simulink library "EmE_MBD_Blockset"  (R2018a)
settings: Solver=ode1  StartTime=0.0  StopTime=Inf  FixedStep=0.001  RelTol=1e-3  EnableMultiTasking=on
PostLoadFcn:
  | , if any(exist('dsrtsu_mdlpostloadfcn', 'file') == [2, 3, 6]), try dsrtsu_mdlpostloadfcn('Execute', bdroot); catch fprintf('Error in PostLoadFcn (dsrtsu_mdlpostloadfcn) for model "%s":\n %s\n', bdroot, lasterr); end, end,
undefined symbols (not defined in the file or in its folder): ENUM_TSC1_CONTROL_PURPOSE_T, gcbh, GLB_SWITCH_T
libraries: simulink x237, $bdroot x115, simulink_need_slupdate x26, MotoHawk_lib x13, simulink_extras x3
(part 4 of 11)

== system EmE_MBD_Blockset/Math Operators/Normalize_on_min_max ==
  Max : Inport
  In : Inport  Port=2
  Min : Inport  Port=3
  Constant : Constant  Value=true
  Divide1 : Product  Inputs=*/  InputSameDT=on
  Divide2 : Product  Inputs=*/  InputSameDT=on
  Dynamic_saturation : $bdroot/Discontinuities/Dynamic_saturation
  If_Then_Else : $bdroot/Signal Routing/If_Then_Else
  Subtract1 : Sum  Inputs=+-  InputSameDT=on
  Subtract3 : Sum  Inputs=+-  InputSameDT=on
  Subtract4 : Sum  Inputs=-+  InputSameDT=on
  Norm : Outport  LibraryBlock=$bdroot/Sinks/Out  OutputWhenDisabled=reset
  wires:
  Dynamic_saturation/1 -> Subtract1/2, Subtract3/1
  Max/1 -> Dynamic_saturation/1, Subtract4/2, Subtract1/1
  Min/1 -> Dynamic_saturation/3, Subtract4/1, Subtract3/2
  Subtract1/1 -> Divide1/1
  Subtract4/1 -> Divide1/2, Divide2/2
  In/1 -> Dynamic_saturation/2
  Subtract3/1 -> Divide2/1
  Constant/1 -> If_Then_Else/1
  Divide2/1 -> If_Then_Else/2  "norm_on_min"
  Divide1/1 -> If_Then_Else/3  "norm_on_max"
  If_Then_Else/1 -> Norm/1

== system EmE_MBD_Blockset/Math Operators/Slew ==
  In : Inport
  Inc : Inport  Port=2
  Dec : Inport  Port=3
  dT : Inport  Port=4
  Abs : $bdroot/Math Operators/Abs
  Abs1 : $bdroot/Math Operators/Abs
  Add1 : Sum  InputSameDT=on
  Check Static Lower Bound : simulink/Model Verification/Check Static  Lower Bound  Description=0 <= u  min=0  min_included=on  enabled=on  stopWhenAssertionFail=on  export=off  icon=graphic
      settings: SourceProductName=Simulink
  MinMax1 : MinMax  Function=max  Inputs=2  InputSameDT=on
  MinMax2 : MinMax  Inputs=2  InputSameDT=on
  Product1 : Product  InputSameDT=on
  Product2 : Product  InputSameDT=on
  Subtract1 : Sum  Inputs=+-  InputSameDT=on
  Unit Delay External IC : simulink_need_slupdate/Unit Delay External IC  tsamp=-1
      settings: SourceProductName=Simulink  SourceProductBaseCode=SL
  Out : Outport
  wires:
  Add1/1 -> MinMax2/2
  Subtract1/1 -> MinMax1/2
  MinMax1/1 -> Out/1, Unit Delay External IC/1
  Product1/1 -> Add1/2
  Unit Delay External IC/1 -> Subtract1/1, Add1/1
  Dec/1 -> Abs1/1
  MinMax2/1 -> MinMax1/1
  Inc/1 -> Check Static Lower Bound/1, Abs/1
  In/1 -> MinMax2/1, Unit Delay External IC/2
  Product2/1 -> Subtract1/2
  Abs/1 -> Product1/1
  Abs1/1 -> Product2/2
  dT/1 -> Product2/1, Product1/2

== system EmE_MBD_Blockset/Math Operators/Slew_at_event ==
  F_Event_trigger : Inport
  Init : Inport  Port=2
  In : Inport  Port=3
  Inc : Inport  Port=4
  Dec : Inport  Port=5
  dT : Inport  Port=6
  Enable : EnablePort  StatesWhenEnabling=reset
  Abs : Abs
  Constant1 : Constant
  RS flip-flop : $bdroot/Logic and Bit Operations/RS flip-flop
  Relational Operator1 : $bdroot/Logic and Bit Operations/Relational Operator  func=<=
  Rising_edge : $bdroot/Discontinuities/Rising_edge  initact=off
      settings: AttributesFormatString=Action on IC: %<initact>
  Slew_init_reset : $bdroot/Math Operators/Slew_init_reset
  Subtract : Sum  Inputs=-+  InputSameDT=on
  Terminator : Terminator
  F_Out_slewing : Outport  OutputWhenDisabled=reset  InitialOutput=false
      settings: AttributesFormatString=IC: %<InitialOutput>\nDisabled value: %<OutputWhenDisabled>
  Out : Outport  Port=2  OutputWhenDisabled=reset  InitialOutput=single(0)
      settings: AttributesFormatString=IC: %<InitialOutput>\nDisabled value: %<OutputWhenDisabled>
  wires:
  RS flip-flop/2 -> Terminator/1
  RS flip-flop/1 -> F_Out_slewing/1  "F_Value_slew_enabled"
  Relational Operator1/1 -> RS flip-flop/1
  Constant1/1 -> Relational Operator1/2
  Subtract/1 -> Abs/1
  Abs/1 -> Relational Operator1/1
  In/1 -> Slew_init_reset/3, Subtract/2
  Init/1 -> Slew_init_reset/2
  Rising_edge/1 -> Slew_init_reset/1
  F_Event_trigger/1 -> Rising_edge/1, RS flip-flop/2
  dT/1 -> Slew_init_reset/6
  Dec/1 -> Slew_init_reset/5
  Inc/1 -> Slew_init_reset/4
  Slew_init_reset/1 -> Subtract/1, Out/1  "Value_slewed"

== system EmE_MBD_Blockset/Math Operators/Slew_init_reset ==
  F_Reset : Inport
  Init : Inport  Port=2
  In : Inport  Port=3
  Inc : Inport  Port=4
  Dec : Inport  Port=5
  dT : Inport  Port=6
  Abs : $bdroot/Math Operators/Abs
  Abs1 : $bdroot/Math Operators/Abs
  Add1 : Sum  InputSameDT=on
  Check Static Lower Bound : simulink/Model Verification/Check Static  Lower Bound  Description=0 <= u  min=0  min_included=on  enabled=on  stopWhenAssertionFail=on  export=off  icon=graphic
      settings: SourceProductName=Simulink
  Constant : Constant  Value=false
  If_Then_Else : $bdroot/Signal Routing/If_Then_Else
  Logical Operator1 : $bdroot/Logic and Bit Operations/Logical Operator  Operator=OR  Inputs=2
  MinMax1 : MinMax  Function=max  Inputs=2  InputSameDT=on
  MinMax2 : MinMax  Inputs=2  InputSameDT=on
  Product1 : Product  InputSameDT=on
  Product2 : Product  InputSameDT=on
  Subtract1 : Sum  Inputs=+-  InputSameDT=on
  Unit Delay External IC : simulink_need_slupdate/Unit Delay External IC  tsamp=-1
      settings: SourceProductName=Simulink  SourceProductBaseCode=SL
  Unit_Delay : UnitDelay  InitialCondition=true  SampleTime=-1
      settings: AttributesFormatString=IC: %<vinit>
  Out : Outport
  wires:
  MinMax2/1 -> MinMax1/1
  Product1/1 -> Add1/2
  MinMax1/1 -> If_Then_Else/3
  In/1 -> MinMax2/1, Unit Delay External IC/2
  Product2/1 -> Subtract1/2
  Add1/1 -> MinMax2/2
  Subtract1/1 -> MinMax1/2
  Unit Delay External IC/1 -> Subtract1/1, Add1/1
  Inc/1 -> Check Static Lower Bound/1, Abs/1
  Dec/1 -> Abs1/1
  dT/1 -> Product2/1, Product1/2
  Unit_Delay/1 -> Logical Operator1/2
  Init/1 -> If_Then_Else/2
  F_Reset/1 -> Logical Operator1/1
  Logical Operator1/1 -> If_Then_Else/1
  If_Then_Else/1 -> Unit Delay External IC/1, Out/1
  Constant/1 -> Unit_Delay/1
  Abs1/1 -> Product2/2
  Abs/1 -> Product1/1

== system EmE_MBD_Blockset/Math Operators/Slope_intercept ==
  X1 : Inport
  X2 : Inport  Port=2
  Y1 : Inport  Port=3
  Y2 : Inport  Port=4
  Compare To Zero : simulink/Logic and Bit Operations/Compare To Zero  relop===  OutDataTypeStr=boolean
  Constant10 : Constant  Value=0.0001
  Divide : Product  Inputs=*/  InputSameDT=on
  If_Then_Else : $bdroot/Signal Routing/If_Then_Else
  Product : Product  InputSameDT=on
  Subtract : Sum  Inputs=+-  InputSameDT=on
  Subtract1 : Sum  Inputs=+-  InputSameDT=on
  Subtract2 : Sum  Inputs=+-  InputSameDT=on
  m : Outport  OutputWhenDisabled=reset  InitialOutput=0
  b : Outport  Port=2  OutputWhenDisabled=reset  InitialOutput=0
  wires:
  Subtract2/1 -> b/1
  Divide/1 -> Product/1, m/1
  Subtract/1 -> Divide/1
  Subtract1/1 -> If_Then_Else/3, Compare To Zero/1
  Product/1 -> Subtract2/2
  Y2/1 -> Subtract/1
  X1/1 -> Subtract1/2, Product/2
  Y1/1 -> Subtract/2, Subtract2/1
  X2/1 -> Subtract1/1
  Compare To Zero/1 -> If_Then_Else/1
  Constant10/1 -> If_Then_Else/2
  If_Then_Else/1 -> Divide/2

== system EmE_MBD_Blockset/Math Operators/Soft_transition ==
  In : Inport
  T_Inc : Inport  Port=2
  T_Dec : Inport  Port=3
  Abs2 : $bdroot/Math Operators/Abs
  CPV : $bdroot/Sources/CPV  conval=false
  Detect Change : simulink/Logic and Bit Operations/Detect Change  vinit=0  InputProcessing=Inherited  OutDataTypeStr=boolean
      settings: AttributesFormatString=IC: %<vinit>
  Divide1 : Product  Inputs=*/  InputSameDT=on
  Divide2 : Product  Inputs=*/  InputSameDT=on
  If_Then_Else2 : $bdroot/Signal Routing/If_Then_Else
  If_Then_Else3 : $bdroot/Signal Routing/If_Then_Else
  MinMax : MinMax  Function=max  Inputs=2  InputSameDT=on
  MinMax1 : MinMax  Function=max  Inputs=2  InputSameDT=on
  Saturation : Saturate  UpperLimit=Inf  LowerLimit=0.0001
      settings: AttributesFormatString=%<LowerLimit>-%<UpperLimit>
  Saturation1 : Saturate  UpperLimit=Inf  LowerLimit=0.0001
      settings: AttributesFormatString=%<LowerLimit>-%<UpperLimit>
  Slew_init_reset : $bdroot/Math Operators/Slew_init_reset
  Subtract : Sum  Inputs=+-  InputSameDT=on
  Unit Delay External IC2 : simulink_need_slupdate/Unit Delay External IC  tsamp=-1
      settings: SourceProductName=Simulink  SourceProductBaseCode=SL
  Unit Delay External IC3 : simulink_need_slupdate/Unit Delay External IC  tsamp=-1
      settings: SourceProductName=Simulink  SourceProductBaseCode=SL
  Unit_Delay : UnitDelay  SampleTime=-1
      settings: AttributesFormatString=IC: %<vinit>
  dT : $bdroot/Sources/dT
  Out : Outport  OutputWhenDisabled=reset
  wires:
  Slew_init_reset/1 -> Unit_Delay/1, Out/1
  CPV/1 -> Slew_init_reset/1
  dT/1 -> MinMax1/2, MinMax/2, Slew_init_reset/6
  Unit_Delay/1 -> [Out_prev]
  In/1 -> Slew_init_reset/3, Slew_init_reset/2, Detect Change/1, Subtract/2
  [Out_prev] -> Subtract/1
  Subtract/1 -> Abs2/1  "err"
  Detect Change/1 -> If_Then_Else3/1, If_Then_Else2/1
  Unit Delay External IC3/1 -> If_Then_Else3/3
  Divide1/1 -> Unit Delay External IC3/2, If_Then_Else3/2
  If_Then_Else3/1 -> Slew_init_reset/5, Unit Delay External IC3/1
  T_Inc/1 -> MinMax/1
  Unit Delay External IC2/1 -> If_Then_Else2/3
  Divide2/1 -> Unit Delay External IC2/2, If_Then_Else2/2
  If_Then_Else2/1 -> Unit Delay External IC2/1, Slew_init_reset/4
  Saturation/1 -> Divide2/2
  Saturation1/1 -> Divide1/2
  Abs2/1 -> Divide1/1, Divide2/1  "err_abs"
  MinMax/1 -> Saturation/1
  MinMax1/1 -> Saturation1/1
  T_Dec/1 -> MinMax1/1

== system EmE_MBD_Blockset/Obsolete/Normalize_on_max ==
  Max : Inport
  In : Inport  Port=2
  Min : Inport  Port=3
  Divide1 : Product  Inputs=*/  InputSameDT=on
  Dynamic_saturation : $bdroot/Discontinuities/Dynamic_saturation
  Subtract1 : Sum  Inputs=+-  InputSameDT=on
  Subtract2 : Sum  Inputs=-+  InputSameDT=on
  Norm : Outport  LibraryBlock=$bdroot/Sinks/Out  OutputWhenDisabled=reset
  wires:
  Max/1 -> Subtract1/1, Dynamic_saturation/1, Subtract2/2
  Min/1 -> Subtract2/1, Dynamic_saturation/3
  Divide1/1 -> Norm/1
  Dynamic_saturation/1 -> Subtract1/2
  In/1 -> Dynamic_saturation/2
  Subtract1/1 -> Divide1/1
  Subtract2/1 -> Divide1/2

== system EmE_MBD_Blockset/Obsolete/Normalize_on_min ==
  Max : Inport
  In : Inport  Port=2
  Min : Inport  Port=3
  Divide2 : Product  Inputs=*/  InputSameDT=on
  Dynamic_saturation : $bdroot/Discontinuities/Dynamic_saturation
  Subtract3 : Sum  Inputs=+-  InputSameDT=on
  Subtract4 : Sum  Inputs=-+  InputSameDT=on
  Norm : Outport  LibraryBlock=$bdroot/Sinks/Out  OutputWhenDisabled=reset
  wires:
  In/1 -> Dynamic_saturation/2
  Min/1 -> Dynamic_saturation/3, Subtract4/1, Subtract3/2
  Subtract4/1 -> Divide2/2
  Dynamic_saturation/1 -> Subtract3/1
  Max/1 -> Subtract4/2, Dynamic_saturation/1
  Divide2/1 -> Norm/1
  Subtract3/1 -> Divide2/1

== system EmE_MBD_Blockset/Ports and Subsystems/Enabled Subsystem ==
  In : Inport
  Enable : EnablePort  StatesWhenEnabling=reset
      settings: AttributesFormatString=States when enabling: %<StatesWhenEnabling>
      settings: CopyFcn=|
      | try
      | L = find_system(get(gcbh,'Parent'),'BlockType','Outport');
      | M = find_system(get(gcbh,'Parent'),'BlockType','EnablePort');
      | N = find_system(get(gcbh,'Parent'),'BlockType','TriggerPort');
      | anyoutports = ~isempty(L);
      | anyenableports = ~isempty(M);
      | anytriggerports = ~isempty(N);
      | sys = get_param(L,'Handle');
      | noutports = length(sys);
      | if (anyoutports),
      | for i = 1:noutports,
      | set(sys{i},'AttributesFormatString','IC: %<InitialOutput>\nDisabled value: %<OutputWhenDisabled>')
      | end;
      | end;
      | catch
      | end;
      settings: DeleteFcn=|
      | try
      | L = find_system(get(gcbh,'Parent'),'BlockType','Outport');
      | M = find_system(get(gcbh,'Parent'),'BlockType','EnablePort');
      | N = find_system(get(gcbh,'Parent'),'BlockType','TriggerPort');
      | anyoutports = ~isempty(L);
      | anyenableports = ~isempty(M);
      | anytriggerports = ~isempty(N);
      | sys = get_param(L,'Handle');
      | noutports = length(sys);
      | if ((anyoutports) && (~anytriggerports)),
      | for i = 1:noutports,
      | set(sys{i},'AttributesFormatString','')
      | end;
      | end;
      | catch
      | end;
      settings: NameChangeFcn=|
      | try
      | L = find_system(get(gcbh,'Parent'),'BlockType','Outport');
      | M = find_system(get(gcbh,'Parent'),'BlockType','EnablePort');
      | N = find_system(get(gcbh,'Parent'),'BlockType','TriggerPort');
      | anyoutports = ~isempty(L);
      | anyenableports = ~isempty(M);
      | anytriggerports = ~isempty(N);
      | sys = get_param(L,'Handle');
      | noutports = length(sys);
      | if (anyoutports),
      | for i = 1:noutports,
      | set(sys{i},'AttributesFormatString','IC: %<InitialOutput>\nDisabled value: %<OutputWhenDisabled>')
      | end;
      | end;
      | catch
      | end
      settings: MoveFcn=|
      | try
      | L = find_system(get(gcbh,'Parent'),'BlockType','Outport');
      | M = find_system(get(gcbh,'Parent'),'BlockType','EnablePort');
      | N = find_system(get(gcbh,'Parent'),'BlockType','TriggerPort');
      | anyoutports = ~isempty(L);
      | anyenableports = ~isempty(M);
      | anytriggerports = ~isempty(N);
      | sys = get_param(L,'Handle');
      | noutports = length(sys);
      | if (anyoutports),
      | for i = 1:noutports,
      | set(sys{i},'AttributesFormatString','IC: %<InitialOutput>\nDisabled value: %<OutputWhenDisabled>')
      | end;
      | end;
      | catch
      | end;
  Out : Outport  LibraryBlock=$bdroot/Sinks/Out  OutputWhenDisabled=reset
      settings: AttributesFormatString=IC: %<InitialOutput>\nDisabled value: %<OutputWhenDisabled>
  wires:
  In/1 -> Out/1

== system EmE_MBD_Blockset/Ports and Subsystems/Enabled and Triggered Subsystem ==
  In : Inport
  Enable : EnablePort  StatesWhenEnabling=reset
      settings: AttributesFormatString=States when enabling: %<StatesWhenEnabling>
      settings: CopyFcn=|
      | try
      | L = find_system(get(gcbh,'Parent'),'BlockType','Outport');
      | M = find_system(get(gcbh,'Parent'),'BlockType','EnablePort');
      | N = find_system(get(gcbh,'Parent'),'BlockType','TriggerPort');
      | anyoutports = ~isempty(L);
      | anyenableports = ~isempty(M);
      | anytriggerports = ~isempty(N);
      | sys = get_param(L,'Handle');
      | noutports = length(sys);
      | if (anyoutports),
      | for i = 1:noutports,
      | set(sys{i},'AttributesFormatString','IC: %<InitialOutput>\nDisabled value: %<OutputWhenDisabled>')
      | end;
      | end;
      | catch
      | end;
      settings: DeleteFcn=|
      | try
      | L = find_system(get(gcbh,'Parent'),'BlockType','Outport');
      | M = find_system(get(gcbh,'Parent'),'BlockType','EnablePort');
      | N = find_system(get(gcbh,'Parent'),'BlockType','TriggerPort');
      | anyoutports = ~isempty(L);
      | anyenableports = ~isempty(M);
      | anytriggerports = ~isempty(N);
      | sys = get_param(L,'Handle');
      | noutports = length(sys);
      | if ((anyoutports) && (~anytriggerports)),
      | for i = 1:noutports,
      | set(sys{i},'AttributesFormatString','')
      | end;
      | end;
      | catch
      | end;
      settings: NameChangeFcn=|
      | try
      | L = find_system(get(gcbh,'Parent'),'BlockType','Outport');
      | M = find_system(get(gcbh,'Parent'),'BlockType','EnablePort');
      | N = find_system(get(gcbh,'Parent'),'BlockType','TriggerPort');
      | anyoutports = ~isempty(L);
      | anyenableports = ~isempty(M);
      | anytriggerports = ~isempty(N);
      | sys = get_param(L,'Handle');
      | noutports = length(sys);
      | if (anyoutports),
      | for i = 1:noutports,
      | set(sys{i},'AttributesFormatString','IC: %<InitialOutput>\nDisabled value: %<OutputWhenDisabled>')
      | end;
      | end;
      | catch
      | end
      settings: MoveFcn=|
      | try
      | L = find_system(get(gcbh,'Parent'),'BlockType','Outport');
      | M = find_system(get(gcbh,'Parent'),'BlockType','EnablePort');
      | N = find_system(get(gcbh,'Parent'),'BlockType','TriggerPort');
      | anyoutports = ~isempty(L);
      | anyenableports = ~isempty(M);
      | anytriggerports = ~isempty(N);
      | sys = get_param(L,'Handle');
      | noutports = length(sys);
      | if (anyoutports),
      | for i = 1:noutports,
      | set(sys{i},'AttributesFormatString','IC: %<InitialOutput>\nDisabled value: %<OutputWhenDisabled>')
      | end;
      | end;
      | catch
      | end;
  Trigger : TriggerPort  VariantControl=(inherit)
      settings: AttributesFormatString=States when enabling: %<StatesWhenEnabling>
      settings: CopyFcn=|
      | try
      | L = find_system(get(gcbh,'Parent'),'BlockType','Outport');
      | M = find_system(get(gcbh,'Parent'),'BlockType','EnablePort');
      | N = find_system(get(gcbh,'Parent'),'BlockType','TriggerPort');
      | anyoutports = ~isempty(L);
      | anyenableports = ~isempty(M);
      | anytriggerports = ~isempty(N);
      | sys = get_param(L,'Handle');
      | noutports = length(sys);
      | if (anyoutports),
      | for i = 1:noutports,
      | set(sys{i},'AttributesFormatString','IC: %<InitialOutput>\nDisabled value: %<OutputWhenDisabled>')
      | end;
      | end;
      | catch
      | end;
      settings: DeleteFcn=|
      | try
      | L = find_system(get(gcbh,'Parent'),'BlockType','Outport');
      | M = find_system(get(gcbh,'Parent'),'BlockType','EnablePort');
      | N = find_system(get(gcbh,'Parent'),'BlockType','TriggerPort');
      | anyoutports = ~isempty(L);
      | anyenableports = ~isempty(M);
      | anytriggerports = ~isempty(N);
      | sys = get_param(L,'Handle');
      | noutports = length(sys);
      | if ((anyoutports) && (~anyenableports)),
      | for i = 1:noutports,
      | set(sys{i},'AttributesFormatString','')
      | end;
      | end;
      | catch
      | end;
      settings: NameChangeFcn=|
      | try
      | L = find_system(get(gcbh,'Parent'),'BlockType','Outport');
      | M = find_system(get(gcbh,'Parent'),'BlockType','EnablePort');
      | N = find_system(get(gcbh,'Parent'),'BlockType','TriggerPort');
      | anyoutports = ~isempty(L);
      | anyenableports = ~isempty(M);
      | anytriggerports = ~isempty(N);
      | sys = get_param(L,'Handle');
      | noutports = length(sys);
      | if (anyoutports),
      | for i = 1:noutports,
      | set(sys{i},'AttributesFormatString','IC: %<InitialOutput>\nDisabled value: %<OutputWhenDisabled>')
      | end;
      | end;
      | catch
      | end;
      settings: MoveFcn=|
      | try
      | L = find_system(get(gcbh,'Parent'),'BlockType','Outport');
      | M = find_system(get(gcbh,'Parent'),'BlockType','EnablePort');
      | N = find_system(get(gcbh,'Parent'),'BlockType','TriggerPort');
      | anyoutports = ~isempty(L);
      | anyenableports = ~isempty(M);
      | anytriggerports = ~isempty(N);
      | sys = get_param(L,'Handle');
      | noutports = length(sys);
      | if (anyoutports),
      | for i = 1:noutports,
      | set(sys{i},'AttributesFormatString','IC: %<InitialOutput>\nDisabled value: %<OutputWhenDisabled>')
      | end;
      | end;
      | catch
      | end;
  Out : Outport  LibraryBlock=$bdroot/Sinks/Out  OutputWhenDisabled=reset
      settings: AttributesFormatString=IC: %<InitialOutput>\nDisabled value: %<OutputWhenDisabled>
  wires:
  In/1 -> Out/1

== system EmE_MBD_Blockset/Ports and Subsystems/Subsystem ==
  In : Inport
  Out : Outport  LibraryBlock=$bdroot/Sinks/Out  OutputWhenDisabled=reset
  wires:
  In/1 -> Out/1

== system EmE_MBD_Blockset/Ports and Subsystems/Triggered Subsystem ==
  In : Inport
  Trigger : TriggerPort  VariantControl=(inherit)
      settings: AttributesFormatString=States when enabling: %<StatesWhenEnabling>
      settings: CopyFcn=|
      | try
      | L = find_system(get(gcbh,'Parent'),'BlockType','Outport');
      | M = find_system(get(gcbh,'Parent'),'BlockType','EnablePort');
      | N = find_system(get(gcbh,'Parent'),'BlockType','TriggerPort');
      | anyoutports = ~isempty(L);
      | anyenableports = ~isempty(M);
      | anytriggerports = ~isempty(N);
      | sys = get_param(L,'Handle');
      | noutports = length(sys);
      | if (anyoutports),
      | for i = 1:noutports,
      | set(sys{i},'AttributesFormatString','IC: %<InitialOutput>\nDisabled value: %<OutputWhenDisabled>')
      | end;
      | end;
      | catch
      | end;
      settings: DeleteFcn=|
      | try
      | L = find_system(get(gcbh,'Parent'),'BlockType','Outport');
      | M = find_system(get(gcbh,'Parent'),'BlockType','EnablePort');
      | N = find_system(get(gcbh,'Parent'),'BlockType','TriggerPort');
      | anyoutports = ~isempty(L);
      | anyenableports = ~isempty(M);
      | anytriggerports = ~isempty(N);
      | sys = get_param(L,'Handle');
      | noutports = length(sys);
      | if ((anyoutports) && (~anyenableports)),
      | for i = 1:noutports,
      | set(sys{i},'AttributesFormatString','')
      | end;
      | end;
      | catch
      | end;
      settings: NameChangeFcn=|
      | try
      | L = find_system(get(gcbh,'Parent'),'BlockType','Outport');
      | M = find_system(get(gcbh,'Parent'),'BlockType','EnablePort');
      | N = find_system(get(gcbh,'Parent'),'BlockType','TriggerPort');
      | anyoutports = ~isempty(L);
      | anyenableports = ~isempty(M);
      | anytriggerports = ~isempty(N);
      | sys = get_param(L,'Handle');
      | noutports = length(sys);
      | if (anyoutports),
      | for i = 1:noutports,
      | set(sys{i},'AttributesFormatString','IC: %<InitialOutput>\nDisabled value: %<OutputWhenDisabled>')
      | end;
      | end;
      | catch
      | end;
      settings: MoveFcn=|
      | try
      | L = find_system(get(gcbh,'Parent'),'BlockType','Outport');
      | M = find_system(get(gcbh,'Parent'),'BlockType','EnablePort');
      | N = find_system(get(gcbh,'Parent'),'BlockType','TriggerPort');
      | anyoutports = ~isempty(L);
      | anyenableports = ~isempty(M);
      | anytriggerports = ~isempty(N);
      | sys = get_param(L,'Handle');
      | noutports = length(sys);
      | if (anyoutports),
      | for i = 1:noutports,
      | set(sys{i},'AttributesFormatString','IC: %<InitialOutput>\nDisabled value: %<OutputWhenDisabled>')
      | end;
      | end;
      | catch
      | end;
  Out : Outport  LibraryBlock=$bdroot/Sinks/Out  OutputWhenDisabled=reset
      settings: AttributesFormatString=IC: %<InitialOutput>\nDisabled value: %<OutputWhenDisabled>
  wires:
  In/1 -> Out/1

== system EmE_MBD_Blockset/Signal Routing/If_Then_Else ==
  If : Inport
  Then : Inport  Port=2
  Else : Inport  Port=3
  Switch : Switch  Criteria=u2 ~= 0  InputSameDT=on
  Out : Outport
  wires:
  Then/1 -> Switch/1
  Switch/1 -> Out/1
  If/1 -> Switch/2
  Else/1 -> Switch/3

== system EmE_MBD_Blockset/Sources/dT ==
  Digital Clock : DigitalClock  SampleTime=-1
  Subtract : Sum  Inputs=+-  InputSameDT=on
  Unit_Delay : UnitDelay  SampleTime=-1
      settings: AttributesFormatString=IC: %<vinit>
  Out : Outport  OutputWhenDisabled=reset
  wires:
  Digital Clock/1 -> Subtract/1, Unit_Delay/1
  Unit_Delay/1 -> Subtract/2
  Subtract/1 -> Out/1

== system EmE_MBD_Blockset/User-Defined Functions/Compare_VIN_data ==
  VIN_Input_uint8 : Inport  OutDataTypeStr=uint8
  SPN237_VehicleIdentificationNumber : Inport  Port=2  OutDataTypeStr=uint8
  Add1 : Sum  Inputs=+  InputSameDT=on
  Compare To Zero2 : simulink/Logic and Bit Operations/Compare To Zero  relop===  OutDataTypeStr=boolean
  Relational Operator2 : RelationalOperator  Operator=~=  OutDataTypeStr=boolean  RndMeth=Nearest  InputSameDT=on
  F_VIN_Match : Outport
  wires:
  VIN_Input_uint8/1 -> Relational Operator2/1
  Relational Operator2/1 -> Add1/1
  Add1/1 -> Compare To Zero2/1
  Compare To Zero2/1 -> F_VIN_Match/1
  SPN237_VehicleIdentificationNumber/1 -> Relational Operator2/2

== system EmE_MBD_Blockset/User-Defined Functions/Determine_engine_speed_from_vehicle_speed ==
  Transmission_gear_ratio : Inport
  Rear_axle_ratio : Inport  Port=2
  Vehicle_speed_kph : Inport  Port=3
  Tire_diameter_inches : Inport  Port=4
  CONVERSION_CONSTANT_CPV : Constant  Value=63360/(pi*60)
  Constant : Constant  Value=0.01
  Constant2 : Constant  Value=3000
  Divide : Product  Inputs=****/  InputSameDT=on
  KPH_TO_MPH : Gain  Gain=0.6213712  OutDataTypeStr=Inherit: Inherit via back propagation
  MinMax : MinMax  Function=max  Inputs=2  InputSameDT=on
  MinMax1 : MinMax  Inputs=2  InputSameDT=on
  Engine_speed : Outport  OutputWhenDisabled=reset  InitialOutput=single(0)
  wires:
  Divide/1 -> MinMax1/1
  CONVERSION_CONSTANT_CPV/1 -> Divide/4
  Tire_diameter_inches/1 -> MinMax/1
  Vehicle_speed_kph/1 -> KPH_TO_MPH/1
  Transmission_gear_ratio/1 -> Divide/2
  MinMax/1 -> Divide/5
  Constant/1 -> MinMax/2
  MinMax1/1 -> Engine_speed/1  "Engine_speed_target"
  Constant2/1 -> MinMax1/2
  KPH_TO_MPH/1 -> Divide/1
  Rear_axle_ratio/1 -> Divide/3

== system EmE_MBD_Blockset/User-Defined Functions/Determine_permanent_magnet_motor_BEMF_volts_at_magnet_temp ==
  note: BEMF Volts - @ Magnet Temp C @ Input_RPM
  note: BEMF Volts - If magnet temp is at same temp as during ref measurement
  note: This is the Ref RPM that the BEMF voltage measurement was made
  note: This is the BEMF voltage measurement @ Ref RPM
  note: This is the input RPM that you want to determine what the BEMF voltage will be at Magnet Temp C
  note: Neodymium magnet material temperature coefficient 0.11%/degC
  note: Samarium cobalt magnet material temperature coefficient 0.03%/degC
  note: This is the magnet temperature that you want to know what the BEMF voltage will be at Input_RPM
  note: This is the actual magnet temperature during BEMF voltage measurement @ RefRPM
  note: Magnet Temp C = PM Change+AmbTempAtBEMF
      |
      | BEMF Volt =(BEMFAtRefRPM+3)+Step
      |
      | Change = BEMFAtRefRPM-BEMF Volt
      |
      | % Change = Change/BEMFAtRefRPM
      |
      | PM Change = % Change/MagnetMatlCoeff
      |
      | Derived:
      | PM Change = AmbTempAtBEMF - Magnet Temp C
      |
      | % Change/MagnetMatlCoeff = AmbTempAtBEMF - Magnet Temp C
  Magnet_temp_C : Inport
  Magnet_temp_C_at_ref_rpm : Inport  Port=2
  Magnet_matl_temp_coeff_%/degC : Inport  Port=3
  Motor_rpm : Inport  Port=4
  BEMF_voltsAC_at_ref_rpm : Inport  Port=5
  Motor_ref_rpm : Inport  Port=6
  Divide1 : Product  Inputs=**/  InputSameDT=on
  Divide2 : Product  Inputs=**  InputSameDT=on
  Gain : Gain  Gain=0.01
  Product : Product  InputSameDT=on
  Subtract : Sum  Inputs=+-  InputSameDT=on
  Subtract1 : Sum  Inputs=-+  InputSameDT=on
  BEMF_voltsAC_ideal : Outport  LibraryBlock=$bdroot/Sinks/Out  OutputWhenDisabled=reset
  BEMF_voltsAC_at_magnet_temp_at_motor_rpm : Outport  LibraryBlock=$bdroot/Sinks/Out  Port=2  OutputWhenDisabled=reset
  wires:
  Magnet_matl_temp_coeff_%/degC/1 -> Product/2
  Subtract1/1 -> BEMF_voltsAC_at_magnet_temp_at_motor_rpm/1
  Magnet_temp_C/1 -> Subtract/1
  Subtract/1 -> Product/1  "PMchange"
  Magnet_temp_C_at_ref_rpm/1 -> Subtract/2
  BEMF_voltsAC_at_ref_rpm/1 -> Divide1/2
  Divide1/1 -> BEMF_voltsAC_ideal/1, Divide2/2, Subtract1/2
  Motor_rpm/1 -> Divide1/1
  Motor_ref_rpm/1 -> Divide1/3
  Gain/1 -> Divide2/1  "PM%change"
  Divide2/1 -> Subtract1/1
  Product/1 -> Gain/1  "%change"

== system EmE_MBD_Blockset/User-Defined Functions/Determine_vehicle_speed_from_trans_output_shaft_speed ==
  SPN191_TransOutputShaftSpeed : Inport
  Rear_axle_ratio : Inport  Port=2
  Tire_diam_inches : Inport  Port=3
  CONVERSION_CONSTANT_CPV1 : Constant  Value=pi
  Divide1 : Product  Inputs=*/  InputSameDT=on
  Divide2 : Product  Inputs=**  InputSameDT=on
  Divide3 : Product  Inputs=**/  InputSameDT=on
  FPM_TO_KPH : Gain  Gain=0.018288  OutDataTypeStr=Inherit: Inherit via back propagation
  Inches_to_feet : Constant  Value=12
  Vehicle_speed : Outport  LibraryBlock=$bdroot/Sinks/Out  OutputWhenDisabled=reset
  wires:
  FPM_TO_KPH/1 -> Vehicle_speed/1  "Vehicle_speed"
  Divide2/1 -> FPM_TO_KPH/1  "Vehicle_speed_feet_per_min"
  Tire_diam_inches/1 -> Divide3/1
  Divide3/1 -> Divide2/2  "Tire_circumference_feet"
  CONVERSION_CONSTANT_CPV1/1 -> Divide3/2
  SPN191_TransOutputShaftSpeed/1 -> Divide1/1
  Rear_axle_ratio/1 -> Divide1/2
  Inches_to_feet/1 -> Divide3/3
  Divide1/1 -> Divide2/1  "Tire_speed_RPM"

== system EmE_MBD_Blockset/User-Defined Functions/Latching_mutual_exclusion ==
  note: This logic will latch output y1 or y2 to TRUE depending on which input (u1 or u2; respectively) goes TRUE first.
      | In the event of a race condition upon start up, both inputs are held low.
  u1 : Inport
  u2 : Inport  Port=2
  CPV : Constant  Value=false
  CPV1 : Constant  Value=false
  Constant : Constant  Value=false
  Constant1 : Constant  Value=false
  If_Then_Else : $bdroot/Signal Routing/If_Then_Else
  If_Then_Else1 : $bdroot/Signal Routing/If_Then_Else
  Logical Operator : Logic  OutDataTypeStr=boolean
  Logical Operator1 : Logic  OutDataTypeStr=boolean
  Logical Operator2 : Logic  OutDataTypeStr=boolean
  Logical Operator4 : Logic  Operator=OR  OutDataTypeStr=boolean
  Logical Operator5 : Logic  Operator=OR  OutDataTypeStr=boolean
  SR flip-flop : $bdroot/Logic and Bit Operations/SR flip-flop
  SR flip-flop1 : $bdroot/Logic and Bit Operations/SR flip-flop
  Unit_Delay{,1..3} (4 alike) : UnitDelay  InitialCondition=true  SampleTime=-1
      settings: AttributesFormatString=IC: %<vinit>
  Unit_Delay4 : UnitDelay  InitialCondition=false  SampleTime=-1
      settings: AttributesFormatString=IC: %<vinit>
  Unit_Delay5 : UnitDelay  InitialCondition=false  SampleTime=-1
      settings: AttributesFormatString=IC: %<vinit>
  y1 : Outport
  y2 : Outport  Port=2
  wires:
  u2/1 -> Logical Operator/2
  Unit_Delay/1 -> Logical Operator4/1
  Constant/1 -> Unit_Delay/1
  Constant1/1 -> Unit_Delay1/1
  SR flip-flop1/2 -> Unit_Delay3/1
  Logical Operator/1 -> SR flip-flop/1
  Logical Operator1/1 -> SR flip-flop1/1
  SR flip-flop/2 -> Unit_Delay2/1
  SR flip-flop1/1 -> If_Then_Else/3, Logical Operator2/1  "F_Truck1841_VIN_Match"
  SR flip-flop/1 -> Logical Operator2/2, If_Then_Else1/3  "F_Truck1842_VIN_Match"
  u1/1 -> Logical Operator1/2
  Logical Operator2/1 -> [f_input_race], If_Then_Else/1, If_Then_Else1/1
  CPV/1 -> If_Then_Else/2
  CPV1/1 -> If_Then_Else1/2
  If_Then_Else1/1 -> y2/1
  If_Then_Else/1 -> y1/1
  Logical Operator4/1 -> SR flip-flop/2
  Unit_Delay4/1 -> Logical Operator4/2
  Unit_Delay2/1 -> [y2_not]
  Unit_Delay3/1 -> [y1_not]
  [y2_not] -> Logical Operator1/1
  [y1_not] -> Logical Operator/1
  Unit_Delay5/1 -> Logical Operator5/2
  Logical Operator5/1 -> SR flip-flop1/2
  Unit_Delay1/1 -> Logical Operator5/1
  [f_input_race] -> Unit_Delay5/1
  [f_input_race] -> Unit_Delay4/1

== system EmE_MBD_Blockset/User-Defined Functions/Snoop ==
  note: Snooped CCP Data Bus
  CAN Receive Slot Trigger1 : MotoHawk_lib/CAN Blocks/CAN Receive Slot Trigger  Tag=Trigger  trig_name=[]  slot='CCP_ATI'  inherited=off  function_name=Trigger_CAN_Slot_CCP_ATI_202705p001
      settings: SourceProductName=MotoHawk
  CAN Receive Slot Trigger15 : MotoHawk_lib/CAN Blocks/CAN Receive Slot Trigger  Tag=Trigger  trig_name=[]  slot='CCP_ETC'  inherited=off  function_name=Trigger_CAN_Slot_CCP_ETC_202705p0011
      settings: SourceProductName=MotoHawk
  CCP_ETC_SS1 : Subsystem  TreatAsAtomicUnit=on
  CCP_ETC_SS2 : Subsystem  TreatAsAtomicUnit=on
  Defaulting : Subsystem  TreatAsAtomicUnit=on
  motohawk_trigger : MotoHawk_lib/Trigger Blocks/motohawk_trigger  Tag=Trigger  trig_name=[]  trigger=FGND_RTI_PERIODIC  priority_order=0  inherited=on  run_disabled=off  override_app_monitor=off  target=GCM_0563_048_0801
      settings: SourceProductName=MotoHawk
  CCP_Data : Outport
  wires:
  motohawk_trigger/1 -> Defaulting/Trigger
  Defaulting/1(CCP_ETC_Data) -> CCP_Data/1
  CCP_ETC_SS2/1(RCV_DATA) -> Defaulting/1(RCV_DATA)
  CCP_ETC_SS1/1(DAQ_Info) -> Defaulting/2(DAQ_Info), CCP_ETC_SS2/1(DAQ_Info)
  CAN Receive Slot Trigger1/1 -> CCP_ETC_SS1/Trigger
  CAN Receive Slot Trigger15/1 -> CCP_ETC_SS2/Trigger

== system EmE_MBD_Blockset/Controllers/Generic_PID_Governor_3/Calculate_PID_terms ==
  F_GPID_reset_gov : Inport
  GPID_control_error : Inport  Port=2
  GPID_dT : Inport  Port=3
  GPID_actual_system_output : Inport  Port=4
  GPID_feed_forward : Inport  Port=5
  GPID_Kp : Inport  Port=6
  GPID_Ki : Inport  Port=7
  GPID_Kd : Inport  Port=8
  GPID_T_filt_d : Inport  Port=9
  F_GPID_aw_cond_integration : Inport  Port=10
  GPID_aw_hysteresis : Inport  Port=11
  F_GPID_aw_hold_i_term : Inport  Port=12
  GPID_output_unlim_prev : Inport  Port=13
  Abs : Abs
  Abs1 : Abs
  Calculate_D_term : Subsystem
  Calculate_I_term : Subsystem
  Calculate_P_term : Subsystem
  Compare To Constant : simulink/Logic and Bit Operations/Compare To Constant  relop=>  const=0.001  OutDataTypeStr=boolean
  Compare To Constant1 : simulink/Logic and Bit Operations/Compare To Constant  relop=>  const=0.001  OutDataTypeStr=boolean
  GPID_p_term : Outport
  GPID_i_term : Outport  Port=2
  GPID_d_term : Outport  Port=3
  F_GPID_hold_i_term : Outport  Port=4
  wires:
  GPID_Kp/1 -> Calculate_P_term/1(GPID_Kp)
  Calculate_P_term/1(GPID_p_term) -> Calculate_I_term/1(GPID_p_term), GPID_p_term/1
  Abs/1 -> Compare To Constant/1
  GPID_actual_system_output/1 -> Calculate_I_term/3(GPID_actual_system_output)
  GPID_feed_forward/1 -> Calculate_I_term/7(GPID_feed_forward)
  GPID_Ki/1 -> Abs/1, Calculate_I_term/2(GPID_Ki)
  F_GPID_aw_cond_integration/1 -> Calculate_I_term/8(F_GPID_aw_cond_integration)
  GPID_aw_hysteresis/1 -> Calculate_I_term/9(GPID_aw_hysteresis)
  F_GPID_aw_hold_i_term/1 -> Calculate_I_term/10(F_GPID_aw_hold_i_term)
  GPID_output_unlim_prev/1 -> Calculate_I_term/11(GPID_output_unlim_prev)
  Calculate_I_term/1(GPID_i_term) -> GPID_i_term/1
  Calculate_I_term/2(F_GPID_hold_i_term) -> F_GPID_hold_i_term/1
  Compare To Constant/1 -> Calculate_I_term/Enable
  Abs1/1 -> Compare To Constant1/1
  Compare To Constant1/1 -> Calculate_D_term/Enable
  GPID_control_error/1 -> Calculate_D_term/4(GPID_control_error), Calculate_I_term/4(GPID_control_error), Calculate_P_term/2(GPID_control_error)
  GPID_dT/1 -> Calculate_D_term/2(GPID_dT), Calculate_I_term/6(GPID_dT)
  Calculate_D_term/1(GPID_d_term) -> GPID_d_term/1
  GPID_Kd/1 -> Abs1/1, Calculate_D_term/1(GPID_Kd)
  GPID_T_filt_d/1 -> Calculate_D_term/5(GPID_T_filt_d)
  F_GPID_reset_gov/1 -> Calculate_D_term/3(F_GPID_reset_gov), Calculate_I_term/5(F_GPID_reset_gov)

== system EmE_MBD_Blockset/Controllers/Generic_PID_Governor_3/Determine_control_error ==
  F_GPID_reset_gov : Inport
  GPID_slew_init : Inport  Port=2
  GPID_setpoint : Inport  Port=3
  GPID_slew_inc_setpoint : Inport  Port=4
  GPID_slew_dec_setpoint : Inport  Port=5
  GPID_dT : Inport  Port=6
  GPID_feedback : Inport  Port=7
  GPID_T_filt_control_error : Inport  Port=8
  LPF_first_order : $bdroot/Discrete/LPF_first_order
  Slew_init_reset : $bdroot/Math Operators/Slew_init_reset
  Subtract : Sum  Inputs=+-  InputSameDT=on
  GPID_control_error : Outport
  wires:
  Subtract/1 -> LPF_first_order/3, LPF_first_order/2
  Slew_init_reset/1 -> Subtract/1
  GPID_slew_inc_setpoint/1 -> Slew_init_reset/4
  GPID_slew_dec_setpoint/1 -> Slew_init_reset/5
  GPID_T_filt_control_error/1 -> LPF_first_order/4
  F_GPID_reset_gov/1 -> Slew_init_reset/1, LPF_first_order/1
  GPID_slew_init/1 -> Slew_init_reset/2
  GPID_setpoint/1 -> Slew_init_reset/3
  GPID_feedback/1 -> Subtract/2
  LPF_first_order/1 -> GPID_control_error/1
  GPID_dT/1 -> Slew_init_reset/6, LPF_first_order/5

== system EmE_MBD_Blockset/Controllers/Generic_PID_Governor_3/Output_PID ==
  GPID_p_term : Inport
  GPID_i_term : Inport  Port=2
  GPID_d_term : Inport  Port=3
  GPID_output_min : Inport  Port=4
  GPID_output_max : Inport  Port=5
  GPID_feed_forward : Inport  Port=6
  Add : Sum  Inputs=++++  InputSameDT=on
  Dynamic_saturation : $bdroot/Discontinuities/Dynamic_saturation
  GPID_output : Outport
  GPID_output_unlim : Outport  Port=2
  wires:
  GPID_d_term/1 -> Add/3
  GPID_output_max/1 -> Dynamic_saturation/1
  GPID_i_term/1 -> Add/2
  Add/1 -> GPID_output_unlim/1, Dynamic_saturation/2
  GPID_feed_forward/1 -> Add/4
  GPID_p_term/1 -> Add/1
  GPID_output_min/1 -> Dynamic_saturation/3
  Dynamic_saturation/1 -> GPID_output/1

== system EmE_MBD_Blockset/Controllers/Generic_PID_Governor_3/Reset_governor ==
  F_GPID_reset : Inport
  Constant : Constant  Value=false
  Logical Operator1 : $bdroot/Logic and Bit Operations/Logical Operator  Operator=OR  Inputs=2
  Unit_Delay : UnitDelay  InitialCondition=true  SampleTime=-1
      settings: AttributesFormatString=IC: %<vinit>
  F_GPID_reset_gov : Outport  OutDataTypeStr=boolean
  wires:
  Unit_Delay/1 -> Logical Operator1/1
  Constant/1 -> Unit_Delay/1
  Logical Operator1/1 -> F_GPID_reset_gov/1
  F_GPID_reset/1 -> Logical Operator1/2

== system EmE_MBD_Blockset/Controllers/Generic_PID_Governor_4/Calculate_PID_terms ==
  F_GPID_reset_gov : Inport
  GPID_control_error : Inport  Port=2
  GPID_dT : Inport  Port=3
  GPID_actual_system_output : Inport  Port=4
  GPID_feed_forward : Inport  Port=5
  GPID_Kp : Inport  Port=6
  GPID_Ki : Inport  Port=7
  GPID_Kd : Inport  Port=8
  GPID_T_filt_d : Inport  Port=9
  F_GPID_aw_cond_integration : Inport  Port=10
  GPID_aw_hysteresis : Inport  Port=11
  F_GPID_aw_hold_i_term : Inport  Port=12
  GPID_output_unlim_prev : Inport  Port=13
  GPID_output_delta : Inport  Port=14
  Abs : Abs
  Abs1 : Abs
  Calculate_D_term : Subsystem
  Calculate_I_term : Subsystem
  Calculate_P_term : Subsystem
  Compare To Constant : simulink/Logic and Bit Operations/Compare To Constant  relop=>  const=0.001  OutDataTypeStr=boolean
  Compare To Constant1 : simulink/Logic and Bit Operations/Compare To Constant  relop=>  const=0.001  OutDataTypeStr=boolean
  GPID_p_term : Outport
  GPID_i_term : Outport  Port=2
  GPID_d_term : Outport  Port=3
  F_GPID_hold_i_term : Outport  Port=4
  wires:
  GPID_Kp/1 -> Calculate_P_term/1(GPID_Kp)
  Calculate_P_term/1(GPID_p_term) -> Calculate_I_term/1(GPID_p_term), GPID_p_term/1
  Abs/1 -> Compare To Constant/1
  GPID_actual_system_output/1 -> Calculate_I_term/3(GPID_actual_system_output)
  GPID_feed_forward/1 -> Calculate_I_term/7(GPID_feed_forward)
  GPID_Ki/1 -> Abs/1, Calculate_I_term/2(GPID_Ki)
  F_GPID_aw_cond_integration/1 -> Calculate_I_term/8(F_GPID_aw_cond_integration)
  GPID_aw_hysteresis/1 -> Calculate_I_term/9(GPID_aw_hysteresis)
  F_GPID_aw_hold_i_term/1 -> Calculate_I_term/10(F_GPID_aw_hold_i_term)
  GPID_output_unlim_prev/1 -> Calculate_I_term/11(GPID_output_unlim_prev)
  Calculate_I_term/1(GPID_i_term) -> GPID_i_term/1
  Calculate_I_term/2(F_GPID_hold_i_term) -> F_GPID_hold_i_term/1
  Compare To Constant/1 -> Calculate_I_term/Enable
  Abs1/1 -> Compare To Constant1/1
  Compare To Constant1/1 -> Calculate_D_term/Enable
  GPID_control_error/1 -> Calculate_D_term/4(GPID_control_error), Calculate_I_term/4(GPID_control_error), Calculate_P_term/2(GPID_control_error)
  GPID_dT/1 -> Calculate_D_term/2(GPID_dT), Calculate_I_term/6(GPID_dT)
  Calculate_D_term/1(GPID_d_term) -> GPID_d_term/1
  GPID_Kd/1 -> Abs1/1, Calculate_D_term/1(GPID_Kd)
  GPID_T_filt_d/1 -> Calculate_D_term/5(GPID_T_filt_d)
  F_GPID_reset_gov/1 -> Calculate_D_term/3(F_GPID_reset_gov), Calculate_I_term/5(F_GPID_reset_gov)
  GPID_output_delta/1 -> Calculate_I_term/12(GPID_output_delta)

== system EmE_MBD_Blockset/Controllers/Generic_PID_Governor_4/Determine_control_error ==
  F_GPID_reset_gov : Inport
  GPID_slew_init : Inport  Port=2
  GPID_setpoint : Inport  Port=3
  GPID_slew_inc_setpoint : Inport  Port=4
  GPID_slew_dec_setpoint : Inport  Port=5
  GPID_dT : Inport  Port=6
  GPID_feedback : Inport  Port=7
  GPID_T_filt_control_error : Inport  Port=8
  LPF_first_order : $bdroot/Discrete/LPF_first_order
  Slew_init_reset : $bdroot/Math Operators/Slew_init_reset
  Subtract : Sum  Inputs=+-  InputSameDT=on
  GPID_control_error : Outport
  wires:
  Subtract/1 -> LPF_first_order/3, LPF_first_order/2
  Slew_init_reset/1 -> Subtract/1
  GPID_slew_inc_setpoint/1 -> Slew_init_reset/4
  GPID_slew_dec_setpoint/1 -> Slew_init_reset/5
  GPID_T_filt_control_error/1 -> LPF_first_order/4
  F_GPID_reset_gov/1 -> Slew_init_reset/1, LPF_first_order/1
  GPID_slew_init/1 -> Slew_init_reset/2
  GPID_setpoint/1 -> Slew_init_reset/3
  GPID_feedback/1 -> Subtract/2
  LPF_first_order/1 -> GPID_control_error/1
  GPID_dT/1 -> Slew_init_reset/6, LPF_first_order/5

== system EmE_MBD_Blockset/Controllers/Generic_PID_Governor_4/Output_PID ==
  GPID_p_term : Inport
  GPID_i_term : Inport  Port=2
  GPID_d_term : Inport  Port=3
  GPID_output_min : Inport  Port=4
  GPID_output_max : Inport  Port=5
  GPID_feed_forward : Inport  Port=6
  Add : Sum  Inputs=++++  InputSameDT=on
  Dynamic_saturation : $bdroot/Discontinuities/Dynamic_saturation
  Subtract : Sum  Inputs=+-  InputSameDT=on
  GPID_output : Outport
  GPID_output_unlim : Outport  Port=2
  GPID_output_delta : Outport  Port=3
  wires:
  GPID_d_term/1 -> Add/3
  GPID_output_max/1 -> Dynamic_saturation/1
  GPID_i_term/1 -> Add/2
  Add/1 -> Subtract/2, GPID_output_unlim/1, Dynamic_saturation/2
  GPID_feed_forward/1 -> Add/4
  GPID_p_term/1 -> Add/1
  GPID_output_min/1 -> Dynamic_saturation/3
  Dynamic_saturation/1 -> Subtract/1, GPID_output/1
  Subtract/1 -> GPID_output_delta/1

== system EmE_MBD_Blockset/Controllers/Generic_PID_Governor_4/Reset_governor ==
  F_GPID_reset : Inport
  Constant : Constant  Value=false
  Logical Operator1 : $bdroot/Logic and Bit Operations/Logical Operator  Operator=OR  Inputs=2
  Unit_Delay : UnitDelay  InitialCondition=true  SampleTime=-1
      settings: AttributesFormatString=IC: %<vinit>
  F_GPID_reset_gov : Outport  OutDataTypeStr=boolean
  wires:
  Unit_Delay/1 -> Logical Operator1/1
  Constant/1 -> Unit_Delay/1
  Logical Operator1/1 -> F_GPID_reset_gov/1
  F_GPID_reset/1 -> Logical Operator1/2

== system EmE_MBD_Blockset/Controllers/PID_saturating_terms/Calculate_D_term ==
  Error : Inport
  D_max : Inport  Port=2
  Kd : Inport  Port=3
  D_min : Inport  Port=4
  dT : Inport  Port=5
  Constant : Constant  Value=false
  Constant1 : Constant  Value=0
  Divide : Product  Inputs=**/  InputSameDT=on
  Dynamic_saturation1 : $bdroot/Discontinuities/Dynamic_saturation
  Subtract3 : Sum  Inputs=+-  InputSameDT=on
  Unit Delay Resettable External IC : simulink_need_slupdate/Unit Delay Resettable External IC  tsamp=-1
      settings: SourceProductName=Simulink  SourceProductBaseCode=SL
  Unit_Delay : UnitDelay  InitialCondition=true  SampleTime=-1
      settings: AttributesFormatString=IC: %<vinit>
  Out : Outport
  wires:
  Subtract3/1 -> Divide/1
  Unit Delay Resettable External IC/1 -> Subtract3/2
  Constant1/1 -> Unit Delay Resettable External IC/3
  dT/1 -> Divide/3
  Divide/1 -> Dynamic_saturation1/2
  Dynamic_saturation1/1 -> Out/1  "d_term"
  Constant/1 -> Unit_Delay/1
  Kd/1 -> Divide/2
  Unit_Delay/1 -> Unit Delay Resettable External IC/2
  Error/1 -> Unit Delay Resettable External IC/1, Subtract3/1
  D_min/1 -> Dynamic_saturation1/3
  D_max/1 -> Dynamic_saturation1/1

== system EmE_MBD_Blockset/Controllers/PID_saturating_terms/Calculate_I_term ==
  Error : Inport
  Output_fb_delta : Inport  Port=2
  dT : Inport  Port=3
  I_max : Inport  Port=4
  Ki : Inport  Port=5
  I_min : Inport  Port=6
  K_fb_delta : Inport  Port=7
  Add : Sum  InputSameDT=on
  Dynamic_saturation2 : $bdroot/Discontinuities/Dynamic_saturation
  Product : Product  InputSameDT=on
  Product1 : Product  InputSameDT=on
  Product2 : Product  InputSameDT=on
  Subtract2 : Sum  Inputs=|++  InputSameDT=on
  Unit_Delay2 : UnitDelay  SampleTime=-1
      settings: AttributesFormatString=IC: %<vinit>
  Unit_Delay3 : UnitDelay  SampleTime=-1
      settings: AttributesFormatString=IC: %<vinit>
  Out : Outport
  Fb_aw : Outport  Port=2
  wires:
  Product/1 -> Subtract2/1
  Unit_Delay2/1 -> Fb_aw/1, Subtract2/2
  Dynamic_saturation2/1 -> Out/1, Unit_Delay3/1  "i_term"
  Product1/1 -> Unit_Delay2/1
  Unit_Delay3/1 -> Add/1
  I_min/1 -> Dynamic_saturation2/3
  Add/1 -> Dynamic_saturation2/2
  Ki/1 -> Product/1
  Output_fb_delta/1 -> Product1/1
  K_fb_delta/1 -> Product1/2
  Product2/1 -> Add/2
  Subtract2/1 -> Product2/2
  Error/1 -> Product/2
  I_max/1 -> Dynamic_saturation2/1
  dT/1 -> Product2/1

== system EmE_MBD_Blockset/Controllers/PID_saturating_terms/Calculate_P_term ==
  P_max : Inport
  Kp : Inport  Port=2
  Error : Inport  Port=3
  P_min : Inport  Port=4
  Dynamic_saturation : $bdroot/Discontinuities/Dynamic_saturation
  Product2 : Product  InputSameDT=on
  Out : Outport
  wires:
  Dynamic_saturation/1 -> Out/1  "p_term"
  Kp/1 -> Product2/1
  Product2/1 -> Dynamic_saturation/2
  Error/1 -> Product2/2
  P_max/1 -> Dynamic_saturation/1
  P_min/1 -> Dynamic_saturation/3

== system EmE_MBD_Blockset/Discontinuities/Debounce/Debounce_timers ==
  F_In : Inport
  On_timer_T_secs : Inport  Port=2
  Off_timer_T_secs : Inport  Port=3
  CPV1 : Constant  Value=0
  CPV8 : Constant  Value=0
  Compare To Zero1 : simulink/Logic and Bit Operations/Compare To Zero  relop=<=  OutDataTypeStr=boolean
  Compare To Zero2 : simulink/Logic and Bit Operations/Compare To Zero  relop=<=  OutDataTypeStr=boolean
  Logical Operator : $bdroot/Logic and Bit Operations/Logical Operator  Operator=NOT  Inputs=2
  Rising_edge1 : $bdroot/Discontinuities/Rising_edge  initact=off
      settings: AttributesFormatString=Action on IC: %<initact>
  Rising_edge2 : $bdroot/Discontinuities/Rising_edge  initact=off
      settings: AttributesFormatString=Action on IC: %<initact>
  Terminator1 : Terminator
  Terminator2 : Terminator
  Timer_enabled_with_reset : $bdroot/Discrete/Timer_enabled_with_reset
  Timer_enabled_with_reset1 : $bdroot/Discrete/Timer_enabled_with_reset
  dT : $bdroot/Sources/dT
  F_On_timer_complete : Outport  LibraryBlock=$bdroot/Sinks/Out  OutputWhenDisabled=reset
  F_Off_timer_complete : Outport  LibraryBlock=$bdroot/Sinks/Out  Port=2  OutputWhenDisabled=reset
  wires:
  Timer_enabled_with_reset1/2 -> Compare To Zero1/1
  Compare To Zero1/1 -> F_Off_timer_complete/1
  Timer_enabled_with_reset1/1 -> Terminator1/1
  dT/1 -> Timer_enabled_with_reset1/5, Timer_enabled_with_reset/5
  Compare To Zero2/1 -> F_On_timer_complete/1
  CPV1/1 -> Timer_enabled_with_reset1/3
  Rising_edge1/1 -> Timer_enabled_with_reset1/2
  Off_timer_T_secs/1 -> Timer_enabled_with_reset1/4
  On_timer_T_secs/1 -> Timer_enabled_with_reset/4
  Rising_edge2/1 -> Timer_enabled_with_reset/2
  F_In/1 -> Logical Operator/1, Rising_edge2/1, Timer_enabled_with_reset/1
  Timer_enabled_with_reset/1 -> Terminator2/1
  CPV8/1 -> Timer_enabled_with_reset/3
  Timer_enabled_with_reset/2 -> Compare To Zero2/1
  Logical Operator/1 -> Timer_enabled_with_reset1/1, Rising_edge1/1

== system EmE_MBD_Blockset/Discrete/DT1_Derivative_lag/Cubic_Approximation ==
  In1 : Inport
  Add2 : Sum  Inputs=++++  InputSameDT=on
  Constant2 : Constant
  Product{4..8} (5 alike) : Product  InputSameDT=on
  cubic_appr_x2_factor : Constant  Value=0.468222
  cubic_appr_x3_factor : Constant  Value=0.105562
  cubic_appr_x_factor : Constant  Value=0.995043
  Out1 : Outport
  wires:
  Product7/1 -> Add2/3
  Product6/1 -> Add2/2
  Constant2/1 -> Add2/1
  cubic_appr_x3_factor/1 -> Product8/2
  Add2/1 -> Out1/1
  cubic_appr_x_factor/1 -> Product6/2
  In1/1 -> Product4/1, Product4/2, Product5/2, Product6/1
  Product5/1 -> Product8/1
  Product4/1 -> Product7/1, Product5/1
  cubic_appr_x2_factor/1 -> Product7/2
  Product8/1 -> Add2/4

== system EmE_MBD_Blockset/Discrete/Discrete-Time Integrator/Integrator_method ==
  note: Forward Euler method:
      | y = y(prev) + K*dT*u(prev)
      |
      | Backward Euler method:
      | y = y(prev) + K*dT*u
      |
      | Trapezoidal method:
      | y = y(prev) + K*dT*[u+u(prev)]/2
  U_in : Inport
  F_Reset : Inport  Port=2
  Add : Sum  InputSameDT=on
  Gain : Gain  Gain=0.5
  Integrator_method : Constant  mask(Constant CPV (EmE)){conval=1}
      mask prompts: conval "Constant value:"
      mask help: Generate a constant value.
      mask init:
      | set_param(gcbh,'Value',conval)
      mask DialogControl DescTextVar Prompt: Constant parameter value.
  Multiport Switch : MultiPortSwitch  DiagnosticForDefault=None  InputSameDT=on
  Unit Delay Resettable External IC : simulink_need_slupdate/Unit Delay Resettable External IC  tsamp=-1
      settings: SourceProductName=Simulink  SourceProductBaseCode=SL
  U_out : Outport  OutputWhenDisabled=reset  InitialOutput=0
  wires:
  U_in/1 -> Unit Delay Resettable External IC/3, Add/2, Unit Delay Resettable External IC/1, Multiport Switch/2  "u_backward_euler"
  Unit Delay Resettable External IC/1 -> Add/1, Multiport Switch/3  "u_forward_euler"
  Add/1 -> Gain/1
  Gain/1 -> Multiport Switch/4  "u_trapezoidal"
  Multiport Switch/1 -> U_out/1
  Integrator_method/1 -> Multiport Switch/1
  F_Reset/1 -> Unit Delay Resettable External IC/2

== system EmE_MBD_Blockset/Discrete/Frequency_detector/Triggered Subsystem ==
  In1 : Inport  LatchByDelayingOutsideSignal=on
  Enable : EnablePort
  Trigger : TriggerPort  VariantControl=(inherit)
  Increment Real World : simulink/Additional Math & Discrete/Additional Math: Increment - Decrement/Increment Real World
      settings: SourceProductName=Simulink  SourceProductBaseCode=SL
  Out1 : Outport  OutputWhenDisabled=reset  InitialOutput=0
  wires:
  In1/1 -> Increment Real World/1
  Increment Real World/1 -> Out1/1
